simulink model "RT_01"  (R2018b)
settings: Solver=FixedStepAuto  StartTime=0.0  StopTime=40  FixedStep=0.01  RelTol=1e-3
undefined symbols (not defined in the file): circle, DiscIntNeverNeededParam, Measurement_Computing, National_Instruments, PCI, QUAD04
libraries: sldrtlib x25, simulink x8, simulink_extras x2
(part 1 of 2)
settings Model: ExtModeTrigDuration=120000  Creator=THIEN  LastModifiedBy=TMP
settings SolverCC: AutoInsertRateTranBlk=on  InsertRTBMode=Always
settings DataIOCC: LimitDataPoints=on  MaxDataPoints=25000  SaveFinalState=on  SaveFormat=StructureWithTime  DSMLogging=off  InspectSignalLogs=on  ReturnWorkspaceOutputs=on
settings HardwareCC: TargetLargestAtomicFloat=Float  TargetIntDivRoundTo=Zero  TargetEndianess=LittleEndian  TargetHWDeviceType=Intel->x86-32 (Windows32)
settings RTWCC: SystemTargetFile=sldrtert.tlc  TemplateMakefile=sldrtert.tmf  Description=Simulink Desktop Real-Time (ERT)  RTWCompilerOptimization=on
settings CodeAppCC: MaxIdLength=95
settings SimulinkDesktopRealTimeERTCC: TargetFcnLib=ansi_tfl_table_tmw.mat  TargetLibSuffix=_sldrt.lib  TargetPreCompLibLocation=C:\Program Files\MATLAB\R2018\toolbox\sldrt\lib\win64  GenFloatMathFcnCalls=NOT IN USE  TargetLangStandard=C99 (ISO)  CodeReplacementLibrary=None  UtilityFuncGeneration=Auto  MultiwordTypeDef=System defined  MultiwordLength=2048  DynamicStringBufferSize=256  GenerateFullHeader=on  InferredTypesCompatibility=off  GenerateSampleERTMain=off  GenerateTestInterfaces=off  ModelReferenceCompliant=on  ParMdlRefBuildCompliant=off  CompOptLevelCompliant=on  ConcurrentExecutionCompliant=off  IncludeMdlTerminateFcn=on  GeneratePreprocessorConditionals=Use local settings  CombineOutputUpdateFcns=off  CombineSignalStateStructs=off  GroupInternalDataByFunction=off  SuppressErrorStatus=off  IncludeFileDelimiter=Auto  ERTCustomFileBanners=off  SupportAbsoluteTime=on  LogVarNameModifier=rt_  MatFileLogging=off  MultiInstanceERTCode=off  CodeInterfacePackaging=Nonreusable function  PurelyIntegerCode=off  SupportNonFinite=on  SupportComplex=on  SupportContinuousTime=on  SupportNonInlinedSFcns=on  RemoveDisableFunc=off  RemoveResetFunc=off  SupportVariableSizeSignals=on  ParenthesesLevel=Nominal  CastingMode=Nominal  PreserveStateflowLocalDataDimensions=off  MATLABClassNameForMDSCustomization=Simulink.SoftwareTarget.TargetSpecificTriggerConfigurationBase  ModelStepFunctionPrototypeControlCompliant=off  CPPClassGenCompliant=off  AutosarCompliant=off  MDXCompliant=off  GRTInterface=off  GenerateAllocFcn=off  UseToolchainInfoCompliant=off  GenerateSharedConstants=on  CoderGroups=[]  AccessMethods=[]  LookupTableObjectStructAxisOrder=1,2,3,4,...  LUTObjectStructOrderExplicitValues=Size,Breakpoints,Table  LUTObjectStructOrderEvenSpacing=Size,Breakpoints,Table  ArrayLayout=Column-major  UnsupportedSFcnMsg=error  ERTHeaderFileRootName=$R$E  ERTSourceFileRootName=$R$E  ERTDataFileRootName=$R_data  GenerateASAP2=off  DSAsUniqueAccess=off  InlinedParameterPlacement=Hierarchical  TargetOS=BareBoardExample  MultiInstanceErrorCode=Error  RootIOFormat=Individual arguments  RTWCAPISignals=off  RTWCAPIParams=off  RTWCAPIStates=off  RTWCAPIRootIO=off  ERTSrcFileBannerTemplate=ert_code_template.cgt  ERTHdrFileBannerTemplate=ert_code_template.cgt  ERTDataSrcFileTemplate=ert_code_template.cgt  ERTDataHdrFileTemplate=ert_code_template.cgt  ERTCustomFileTemplate=example_file_process.tlc  EnableDataOwnership=off  SignalDisplayLevel=10  ParamTuneLevel=10  GlobalDataDefinition=Auto  DataDefinitionFile=global.c  GlobalDataReference=Auto  ERTFilePackagingFormat=Modular  RateTransitionBlockCode=Inline  DataReferenceFile=global.h  PreserveExpressionOrder=off  PreserveIfCondition=off  ConvertIfToSwitch=off  PreserveExternInFcnDecls=on  PreserveStaticInFcnDecls=on  SuppressUnreachableDefaultCases=off  EnableSignedLeftShifts=on  EnableSignedRightShifts=on  IndentStyle=K&R  IndentSize=2  NewlineStyle=Default  EnableUserReplacementTypes=off  MaxIdInt64=MAX_int64_T  MinIdInt64=MIN_int64_T  MaxIdUint64=MAX_uint64_T  MaxIdInt32=MAX_int32_T  MinIdInt32=MIN_int32_T  MaxIdUint32=MAX_uint32_T  MaxIdInt16=MAX_int16_T  MinIdInt16=MIN_int16_T  MaxIdUint16=MAX_uint16_T  MaxIdInt8=MAX_int8_T  MinIdInt8=MIN_int8_T  MaxIdUint8=MAX_uint8_T  BooleanTrueId=true  BooleanFalseId=false  MemSecPackage=--- None ---  MemSecDataConstants=Default  MemSecDataIO=Default  MemSecDataInternal=Default  MemSecDataParameters=Default  MemSecFuncInitTerm=Default  MemSecFuncExecute=Default  MemSecFuncSharedUtil=Default  GroupConstants=Default  GroupRootInputs=Default  GroupRootOutputs=Default  GroupInternal=Default  GroupParameters=Default  GroupDataTransfer=Default  GroupSharedLocalDataStores=Default  GroupInstanceSpecificParameters=Default  GroupModelData=Default  CCListing=off  RebuildAll=off  ExtMode=on  ExtModeTransport=0  ExtModeStaticAlloc=off  ExtModeStaticAllocSize=1000000  ExtModeTesting=off  ExtModeMexFile=sldrtext  ExtModeIntrfLevel=Level1

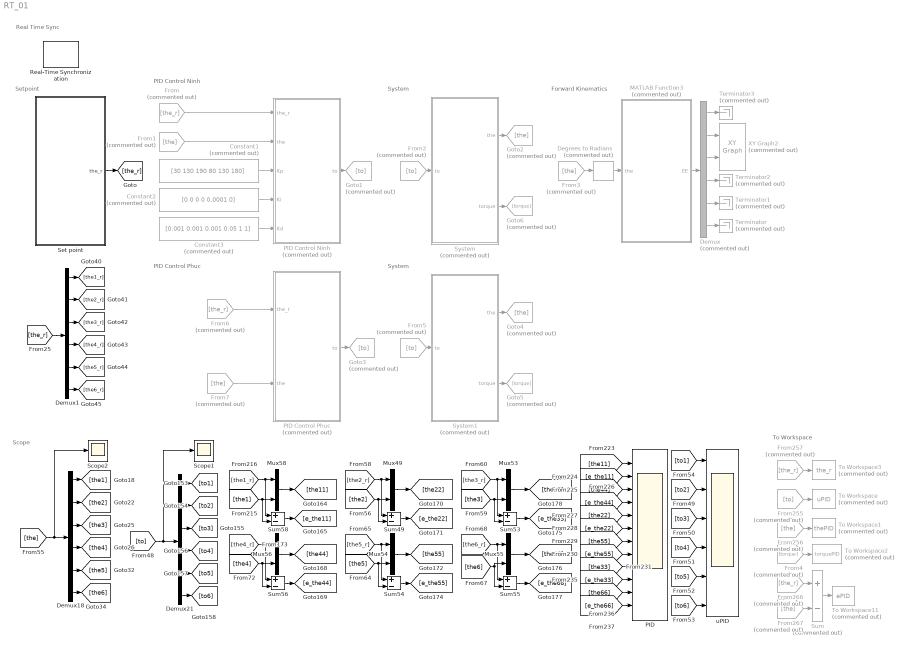
== system RT_01 ==
  note: Real Time Sync
  note: Forward Kinematics
  note: System
  note: PID Control Ninh
  note: Setpoint
  note: Scope
  note: System
  note: PID Control Phuc
  note: To Workspace
  Constant1 : Constant  Commented=on  Value=[30 130 190 80 130 180]
  Constant2 : Constant  Commented=on  Value=[0 0 0 0 0.0001 0]
  Constant3 : Constant  Commented=on  Value=[0.001 0.001 0.001 0.05 1 1]
  Degrees to Radians : simulink_extras/Transformations/Degrees to Radians  Commented=on
  Demux : Demux  Commented=on  Outputs=6
  Demux1 : Demux  Outputs=6
  Demux18 : Demux  Outputs=6
  Demux21 : Demux  Outputs=6
  From{,6,257,266} (4 alike) : From  Commented=on  GotoTag=the_r
  From{1,3,7,256,267} (5 alike) : From  Commented=on  GotoTag=the
  From2 : From  Commented=on  GotoTag=to
  From255 : From  Commented=on  GotoTag=to
  From4 : From  Commented=on  GotoTag=torque
  From5 : From  Commented=on  GotoTag=to
  Goto1 : Goto  Commented=on  GotoTag=to
  Goto2 : Goto  Commented=on  GotoTag=the
  Goto3 : Goto  Commented=on  GotoTag=to
  Goto4 : Goto  Commented=on  GotoTag=the
  Goto5 : Goto  Commented=on  GotoTag=torque
  Goto6 : Goto  Commented=on  GotoTag=torque
  MATLAB Function3 : MATLAB Function  Commented=on  TreatAsAtomicUnit=on
  Mux{49,53..56,58} (6 alike) : Mux  Inputs=2
  PID : Scope  NumInputPorts=12
  PID Control Ninh : Subsystem  Commented=on
  PID Control Phuc : Subsystem  Commented=on
  Real-Time Synchronization : sldrtlib/Real-Time Synchronization  SampleTime=0.01  MaxMissedTicks=10  ShowMissedTicks=off  YieldWhenWaiting=off
  Scope1 : Scope
  Scope2 : Scope
  Set point : Subsystem
  Sum : Sum  Commented=on  Inputs=+-
  Sum{49,53..56,58} (6 alike) : Sum  Inputs=+-
  System : Subsystem  Commented=on
  System1 : Subsystem  Commented=on
  Terminator{,1..3} (4 alike) : Terminator  Commented=on
  To Workspace : ToWorkspace  Commented=on  VariableName=uPID  SaveFormat=Structure With Time  SampleTime=-1
  To Workspace1 : ToWorkspace  Commented=on  VariableName=thePID  SaveFormat=Structure With Time  SampleTime=-1
  To Workspace11 : ToWorkspace  Commented=on  VariableName=ePID  SaveFormat=Structure With Time  SampleTime=-1
  To Workspace2 : ToWorkspace  Commented=on  VariableName=torquePID  SaveFormat=Structure With Time  SampleTime=-1
  To Workspace3 : ToWorkspace  Commented=on  VariableName=the_r  SaveFormat=Structure With Time  SampleTime=-1
  XY Graph2 : simulink/Sinks/XY Graph  Commented=on  xmin=-120  xmax=120  ymin=430  ymax=670  st=-1
  uPID : Scope  NumInputPorts=6
  wires:
  MATLAB Function3/1(EE) -> Demux/1
  Degrees to Radians/1 -> MATLAB Function3/1(the)
  Demux/2 -> XY Graph2/1
  Demux/3 -> XY Graph2/2
  Demux/6 -> Terminator/1
  Demux/5 -> Terminator1/1
  Demux/4 -> Terminator2/1
  Demux/1 -> Terminator3/1
  Constant1/1 -> PID Control Ninh/3(Kp)
  Constant3/1 -> PID Control Ninh/5(Kd)
  Constant2/1 -> PID Control Ninh/4(Ki)
  Set point/1(the_r) -> [the_r]
  From/1 -> PID Control Ninh/1(the_r)
  From1/1 -> PID Control Ninh/2(the)
  PID Control Ninh/1(to) -> Goto1/1
  From2/1 -> System/1(to)
  System/1(the) -> Goto2/1
  From3/1 -> Degrees to Radians/1
  [to2] -> uPID/2
  [to1] -> uPID/1
  [the22] -> PID/5
  [e_the55] -> PID/8
  [e_the66] -> PID/12
  Demux18/6 -> [the6]
  [to5] -> uPID/5
  [e_the22] -> PID/6
  [to3] -> uPID/3
  [the11] -> PID/1
  [the44] -> PID/3
  Mux53/1 -> [the33]
  Mux54/1 -> [the55]
  Sum53/1 -> [e_the33]
  [e_the44] -> PID/4
  [the66] -> PID/11
  Mux49/1 -> [the22]
  [the5] -> Mux54/2, Sum54/2
  Mux56/1 -> [the44]
  Sum58/1 -> [e_the11]
  Demux21/4 -> [to4]
  Sum55/1 -> [e_the66]
  [the1_r] -> Mux58/1, Sum58/1
  Demux18/5 -> [the5]
  [the3] -> Mux53/2, Sum53/2
  Sum49/1 -> [e_the22]
  [the1] -> Mux58/2, Sum58/2
  [the3_r] -> Mux53/1, Sum53/1
  Mux58/1 -> [the11]
  Sum54/1 -> [e_the55]
  [the5_r] -> Mux54/1, Sum54/1
  [the6] -> Mux55/2, Sum55/2
  Sum56/1 -> [e_the44]
  [to] -> Scope1/1, Demux21/1
  Demux21/3 -> [to3]
  [to4] -> uPID/4
  [the4] -> Sum56/2, Mux56/2
  Demux21/2 -> [to2]
  Demux21/6 -> [to6]
  Demux18/4 -> [the4]
  [the4_r] -> Sum56/1, Mux56/1
  Demux18/3 -> [the3]
  [e_the33] -> PID/10
  [e_the11] -> PID/2
  [the6_r] -> Sum55/1, Mux55/1
  [the2] -> Sum49/2, Mux49/2
  [to6] -> uPID/6
  Demux18/2 -> [the2]
  Demux21/5 -> [to5]
  [the33] -> PID/9
  Mux55/1 -> [the66]
  Demux18/1 -> [the1]
  [the55] -> PID/7
  Demux21/1 -> [to1]
  [the2_r] -> Sum49/1, Mux49/1
  Demux1/4 -> [the4_r]
  [the_r] -> Demux1/1
  Demux1/6 -> [the6_r]
  Demux1/3 -> [the3_r]
  Demux1/5 -> [the5_r]
  Demux1/1 -> [the1_r]
  Demux1/2 -> [the2_r]
  PID Control Phuc/1(to) -> Goto3/1
  From6/1 -> PID Control Phuc/1(the_r)
  From7/1 -> PID Control Phuc/2(the)
  System1/1(the) -> Goto4/1
  From5/1 -> System1/1(to)
  [the] -> Scope2/1, Demux18/1
  System1/2(torque) -> Goto5/1
  Sum/1 -> To Workspace11/1
  From266/1 -> Sum/1
  From257/1 -> To Workspace3/1
  From256/1 -> To Workspace1/1
  From267/1 -> Sum/2
  From255/1 -> To Workspace/1
  System/2(torque) -> Goto6/1
  From4/1 -> To Workspace2/1

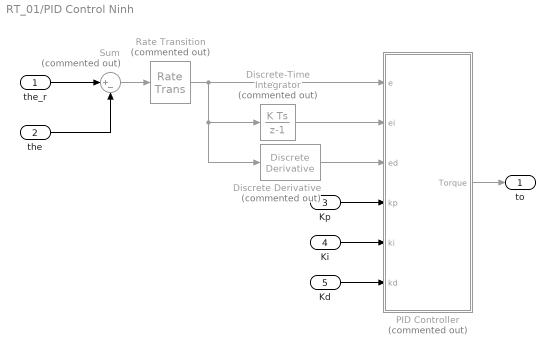
== system RT_01/PID Control Ninh ==
  the_r : Inport
  the : Inport  Port=2
  Kp : Inport  Port=3
  Ki : Inport  Port=4
  Kd : Inport  Port=5
  Discrete Derivative : simulink/Discrete/Discrete Derivative  Commented=on  gainval=1.0  ICPrevScaledInput=0.0  OutMin=[]  OutMax=[]  OutDataType=fixdt(1, 16)  OutScaling=2^-10  DoSatur=off
  Discrete-Time Integrator : DiscreteIntegrator  Commented=on  SampleTime=-1  ICPrevOutput=DiscIntNeverNeededParam  ICPrevScaledInput=DiscIntNeverNeededParam
  PID Controller : MATLAB Function  Commented=on  TreatAsAtomicUnit=on
  Rate Transition : RateTransition  Commented=on  OutPortSampleTime=0.01
  Sum : Sum  Commented=on  Inputs=|+-
  to : Outport
  wires:
  the/1 -> Sum/2
  Ki/1 -> PID Controller/5(ki)
  Discrete Derivative/1 -> PID Controller/3(ed)
  PID Controller/1(Torque) -> to/1
  Rate Transition/1 -> Discrete Derivative/1, Discrete-Time Integrator/1, PID Controller/1(e)
  Kp/1 -> PID Controller/4(kp)
  Kd/1 -> PID Controller/6(kd)
  Discrete-Time Integrator/1 -> PID Controller/2(ei)
  Sum/1 -> Rate Transition/1
  the_r/1 -> Sum/1

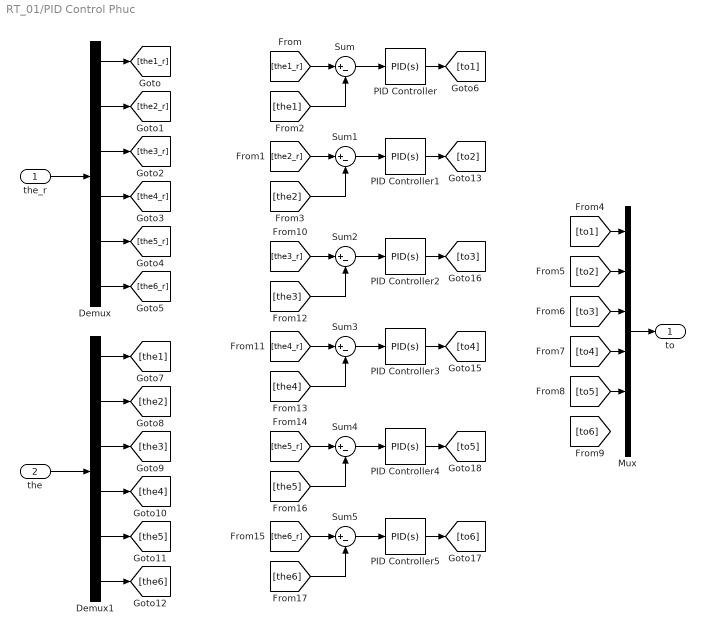
== system RT_01/PID Control Phuc ==
  the_r : Inport
  the : Inport  Port=2
  Demux : Demux  Outputs=6
  Demux1 : Demux  Outputs=6
  Mux : Mux  Inputs=6
  PID Controller : simulink/Continuous/PID Controller  Controller=PID  Form=Parallel  TimeDomain=Continuous-time  SampleTime=0.01  IntegratorMethod=Forward Euler  FilterMethod=Forward Euler  ControllerParametersSource=internal  P=90  I=0  D=4  UseFilter=on  N=100  TunerSelectOption=Transfer Function Based (PID Tuner App)  InitialConditionSource=internal  InitialConditionForIntegrator=0  InitialConditionForFilter=0  DifferentiatorICPrevScaledInput=0  ExternalReset=none  TrackingMode=off  Kt=1  LimitOutput=off  UpperSaturationLimit=inf  LowerSaturationLimit=-inf  LinearizeAsGain=on  AntiWindupMode=none  Kb=1  POutMin=[]  POutMax=[]  IOutMin=[]  IOutMax=[]  DOutMin=[]  DOutMax=[]  NOutMin=[]  NOutMax=[]  SumOutMin=[]  SumOutMax=[]  SaturationOutMin=[]  SaturationOutMax=[]  PParamMin=[]  PParamMax=[]  IParamMin=[]  IParamMax=[]  DParamMin=[]  DParamMax=[]  NParamMin=[]  NParamMax=[]  KbParamMin=[]  KbParamMax=[]  KtParamMin=[]  KtParamMax=[]  KbOutMin=[]  KbOutMax=[]  KtOutMin=[]  KtOutMax=[]  IntegratorOutMin=[]  IntegratorOutMax=[]  FilterOutMin=[]  FilterOutMax=[]  SumI1OutMin=[]  SumI1OutMax=[]  SumI2OutMin=[]  SumI2OutMax=[]  SumI3OutMin=[]  SumI3OutMax=[]  SumI4OutMin=[]  SumI4OutMax=[]  SumDOutMin=[]  SumDOutMax=[]  DifferentiatorOutMin=[]  DifferentiatorOutMax=[]  FilterDiffOutCoefMin=[]  FilterDiffOutCoefMax=[]  ReciprocalOutMin=[]  ReciprocalOutMax=[]  SumDenOutMin=[]  SumDenOutMax=[]  SumNumOutMin=[]  SumNumOutMax=[]  DivideOutMin=[]  DivideOutMax=[]  IntegratorContinuousStateAttributes=''  IntegratorStateMustResolveToSignalObject=off  IntegratorRTWStateStorageClass=Auto  FilterContinuousStateAttributes=''  FilterStateMustResolveToSignalObject=off  FilterRTWStateStorageClass=Auto  ParallelPVariant=InternalParameters  IdealPVariant=Disabled  IVariant=InternalParameters  DVariant=InternalParameters  IntegratorVariant=Continuous  SatVariant=Disabled  AWVariant=Passthrough  PCopyVariant=Disabled  TRVariant=Disabled  FdbkBlocksVariant=Forward  IdealPFdbkVariant=Disabled  SatFdbkVariant=Disabled  DerivativeFilterVariant=ContFilter  NVariant=InternalParameters  NCopyVariant=Disabled  FilterICVariant=InternalICsFilter  IntegratorICVariant=InternalICs  ExternalResetVariant=Disabled  TRSumVariant=Passthrough  SumFdbkVariant=Disabled  SumVariant=Sum_PID
  PID Controller1 : simulink/Continuous/PID Controller  Controller=PID  Form=Parallel  TimeDomain=Continuous-time  SampleTime=0.01  IntegratorMethod=Forward Euler  FilterMethod=Forward Euler  ControllerParametersSource=internal  P=220  I=0  D=12  UseFilter=on  N=100  TunerSelectOption=Transfer Function Based (PID Tuner App)  InitialConditionSource=internal  InitialConditionForIntegrator=0  InitialConditionForFilter=0  DifferentiatorICPrevScaledInput=0  ExternalReset=none  TrackingMode=off  Kt=1  LimitOutput=off  UpperSaturationLimit=inf  LowerSaturationLimit=-inf  LinearizeAsGain=on  AntiWindupMode=none  Kb=1  POutMin=[]  POutMax=[]  IOutMin=[]  IOutMax=[]  DOutMin=[]  DOutMax=[]  NOutMin=[]  NOutMax=[]  SumOutMin=[]  SumOutMax=[]  SaturationOutMin=[]  SaturationOutMax=[]  PParamMin=[]  PParamMax=[]  IParamMin=[]  IParamMax=[]  DParamMin=[]  DParamMax=[]  NParamMin=[]  NParamMax=[]  KbParamMin=[]  KbParamMax=[]  KtParamMin=[]  KtParamMax=[]  KbOutMin=[]  KbOutMax=[]  KtOutMin=[]  KtOutMax=[]  IntegratorOutMin=[]  IntegratorOutMax=[]  FilterOutMin=[]  FilterOutMax=[]  SumI1OutMin=[]  SumI1OutMax=[]  SumI2OutMin=[]  SumI2OutMax=[]  SumI3OutMin=[]  SumI3OutMax=[]  SumI4OutMin=[]  SumI4OutMax=[]  SumDOutMin=[]  SumDOutMax=[]  DifferentiatorOutMin=[]  DifferentiatorOutMax=[]  FilterDiffOutCoefMin=[]  FilterDiffOutCoefMax=[]  ReciprocalOutMin=[]  ReciprocalOutMax=[]  SumDenOutMin=[]  SumDenOutMax=[]  SumNumOutMin=[]  SumNumOutMax=[]  DivideOutMin=[]  DivideOutMax=[]  IntegratorContinuousStateAttributes=''  IntegratorStateMustResolveToSignalObject=off  IntegratorRTWStateStorageClass=Auto  FilterContinuousStateAttributes=''  FilterStateMustResolveToSignalObject=off  FilterRTWStateStorageClass=Auto  ParallelPVariant=InternalParameters  IdealPVariant=Disabled  IVariant=InternalParameters  DVariant=InternalParameters  IntegratorVariant=Continuous  SatVariant=Disabled  AWVariant=Passthrough  PCopyVariant=Disabled  TRVariant=Disabled  FdbkBlocksVariant=Forward  IdealPFdbkVariant=Disabled  SatFdbkVariant=Disabled  DerivativeFilterVariant=ContFilter  NVariant=InternalParameters  NCopyVariant=Disabled  FilterICVariant=InternalICsFilter  IntegratorICVariant=InternalICs  ExternalResetVariant=Disabled  TRSumVariant=Passthrough  SumFdbkVariant=Disabled  SumVariant=Sum_PID
  PID Controller2 : simulink/Continuous/PID Controller  Controller=PID  Form=Parallel  TimeDomain=Continuous-time  SampleTime=0.01  IntegratorMethod=Forward Euler  FilterMethod=Forward Euler  ControllerParametersSource=internal  P=270  I=0  D=12  UseFilter=on  N=100  TunerSelectOption=Transfer Function Based (PID Tuner App)  InitialConditionSource=internal  InitialConditionForIntegrator=0  InitialConditionForFilter=0  DifferentiatorICPrevScaledInput=0  ExternalReset=none  TrackingMode=off  Kt=1  LimitOutput=off  UpperSaturationLimit=inf  LowerSaturationLimit=-inf  LinearizeAsGain=on  AntiWindupMode=none  Kb=1  POutMin=[]  POutMax=[]  IOutMin=[]  IOutMax=[]  DOutMin=[]  DOutMax=[]  NOutMin=[]  NOutMax=[]  SumOutMin=[]  SumOutMax=[]  SaturationOutMin=[]  SaturationOutMax=[]  PParamMin=[]  PParamMax=[]  IParamMin=[]  IParamMax=[]  DParamMin=[]  DParamMax=[]  NParamMin=[]  NParamMax=[]  KbParamMin=[]  KbParamMax=[]  KtParamMin=[]  KtParamMax=[]  KbOutMin=[]  KbOutMax=[]  KtOutMin=[]  KtOutMax=[]  IntegratorOutMin=[]  IntegratorOutMax=[]  FilterOutMin=[]  FilterOutMax=[]  SumI1OutMin=[]  SumI1OutMax=[]  SumI2OutMin=[]  SumI2OutMax=[]  SumI3OutMin=[]  SumI3OutMax=[]  SumI4OutMin=[]  SumI4OutMax=[]  SumDOutMin=[]  SumDOutMax=[]  DifferentiatorOutMin=[]  DifferentiatorOutMax=[]  FilterDiffOutCoefMin=[]  FilterDiffOutCoefMax=[]  ReciprocalOutMin=[]  ReciprocalOutMax=[]  SumDenOutMin=[]  SumDenOutMax=[]  SumNumOutMin=[]  SumNumOutMax=[]  DivideOutMin=[]  DivideOutMax=[]  IntegratorContinuousStateAttributes=''  IntegratorStateMustResolveToSignalObject=off  IntegratorRTWStateStorageClass=Auto  FilterContinuousStateAttributes=''  FilterStateMustResolveToSignalObject=off  FilterRTWStateStorageClass=Auto  ParallelPVariant=InternalParameters  IdealPVariant=Disabled  IVariant=InternalParameters  DVariant=InternalParameters  IntegratorVariant=Continuous  SatVariant=Disabled  AWVariant=Passthrough  PCopyVariant=Disabled  TRVariant=Disabled  FdbkBlocksVariant=Forward  IdealPFdbkVariant=Disabled  SatFdbkVariant=Disabled  DerivativeFilterVariant=ContFilter  NVariant=InternalParameters  NCopyVariant=Disabled  FilterICVariant=InternalICsFilter  IntegratorICVariant=InternalICs  ExternalResetVariant=Disabled  TRSumVariant=Passthrough  SumFdbkVariant=Disabled  SumVariant=Sum_PID
  PID Controller3 : simulink/Continuous/PID Controller  Controller=PID  Form=Parallel  TimeDomain=Continuous-time  SampleTime=0.01  IntegratorMethod=Forward Euler  FilterMethod=Forward Euler  ControllerParametersSource=internal  P=110  I=0  D=6  UseFilter=on  N=100  TunerSelectOption=Transfer Function Based (PID Tuner App)  InitialConditionSource=internal  InitialConditionForIntegrator=0  InitialConditionForFilter=0  DifferentiatorICPrevScaledInput=0  ExternalReset=none  TrackingMode=off  Kt=1  LimitOutput=off  UpperSaturationLimit=inf  LowerSaturationLimit=-inf  LinearizeAsGain=on  AntiWindupMode=none  Kb=1  POutMin=[]  POutMax=[]  IOutMin=[]  IOutMax=[]  DOutMin=[]  DOutMax=[]  NOutMin=[]  NOutMax=[]  SumOutMin=[]  SumOutMax=[]  SaturationOutMin=[]  SaturationOutMax=[]  PParamMin=[]  PParamMax=[]  IParamMin=[]  IParamMax=[]  DParamMin=[]  DParamMax=[]  NParamMin=[]  NParamMax=[]  KbParamMin=[]  KbParamMax=[]  KtParamMin=[]  KtParamMax=[]  KbOutMin=[]  KbOutMax=[]  KtOutMin=[]  KtOutMax=[]  IntegratorOutMin=[]  IntegratorOutMax=[]  FilterOutMin=[]  FilterOutMax=[]  SumI1OutMin=[]  SumI1OutMax=[]  SumI2OutMin=[]  SumI2OutMax=[]  SumI3OutMin=[]  SumI3OutMax=[]  SumI4OutMin=[]  SumI4OutMax=[]  SumDOutMin=[]  SumDOutMax=[]  DifferentiatorOutMin=[]  DifferentiatorOutMax=[]  FilterDiffOutCoefMin=[]  FilterDiffOutCoefMax=[]  ReciprocalOutMin=[]  ReciprocalOutMax=[]  SumDenOutMin=[]  SumDenOutMax=[]  SumNumOutMin=[]  SumNumOutMax=[]  DivideOutMin=[]  DivideOutMax=[]  IntegratorContinuousStateAttributes=''  IntegratorStateMustResolveToSignalObject=off  IntegratorRTWStateStorageClass=Auto  FilterContinuousStateAttributes=''  FilterStateMustResolveToSignalObject=off  FilterRTWStateStorageClass=Auto  ParallelPVariant=InternalParameters  IdealPVariant=Disabled  IVariant=InternalParameters  DVariant=InternalParameters  IntegratorVariant=Continuous  SatVariant=Disabled  AWVariant=Passthrough  PCopyVariant=Disabled  TRVariant=Disabled  FdbkBlocksVariant=Forward  IdealPFdbkVariant=Disabled  SatFdbkVariant=Disabled  DerivativeFilterVariant=ContFilter  NVariant=InternalParameters  NCopyVariant=Disabled  FilterICVariant=InternalICsFilter  IntegratorICVariant=InternalICs  ExternalResetVariant=Disabled  TRSumVariant=Passthrough  SumFdbkVariant=Disabled  SumVariant=Sum_PID
  PID Controller4 : simulink/Continuous/PID Controller  Controller=PID  Form=Parallel  TimeDomain=Continuous-time  SampleTime=0.01  IntegratorMethod=Forward Euler  FilterMethod=Forward Euler  ControllerParametersSource=internal  P=150  I=0  D=4  UseFilter=on  N=100  TunerSelectOption=Transfer Function Based (PID Tuner App)  InitialConditionSource=internal  InitialConditionForIntegrator=0  InitialConditionForFilter=0  DifferentiatorICPrevScaledInput=0  ExternalReset=none  TrackingMode=off  Kt=1  LimitOutput=off  UpperSaturationLimit=inf  LowerSaturationLimit=-inf  LinearizeAsGain=on  AntiWindupMode=none  Kb=1  POutMin=[]  POutMax=[]  IOutMin=[]  IOutMax=[]  DOutMin=[]  DOutMax=[]  NOutMin=[]  NOutMax=[]  SumOutMin=[]  SumOutMax=[]  SaturationOutMin=[]  SaturationOutMax=[]  PParamMin=[]  PParamMax=[]  IParamMin=[]  IParamMax=[]  DParamMin=[]  DParamMax=[]  NParamMin=[]  NParamMax=[]  KbParamMin=[]  KbParamMax=[]  KtParamMin=[]  KtParamMax=[]  KbOutMin=[]  KbOutMax=[]  KtOutMin=[]  KtOutMax=[]  IntegratorOutMin=[]  IntegratorOutMax=[]  FilterOutMin=[]  FilterOutMax=[]  SumI1OutMin=[]  SumI1OutMax=[]  SumI2OutMin=[]  SumI2OutMax=[]  SumI3OutMin=[]  SumI3OutMax=[]  SumI4OutMin=[]  SumI4OutMax=[]  SumDOutMin=[]  SumDOutMax=[]  DifferentiatorOutMin=[]  DifferentiatorOutMax=[]  FilterDiffOutCoefMin=[]  FilterDiffOutCoefMax=[]  ReciprocalOutMin=[]  ReciprocalOutMax=[]  SumDenOutMin=[]  SumDenOutMax=[]  SumNumOutMin=[]  SumNumOutMax=[]  DivideOutMin=[]  DivideOutMax=[]  IntegratorContinuousStateAttributes=''  IntegratorStateMustResolveToSignalObject=off  IntegratorRTWStateStorageClass=Auto  FilterContinuousStateAttributes=''  FilterStateMustResolveToSignalObject=off  FilterRTWStateStorageClass=Auto  ParallelPVariant=InternalParameters  IdealPVariant=Disabled  IVariant=InternalParameters  DVariant=InternalParameters  IntegratorVariant=Continuous  SatVariant=Disabled  AWVariant=Passthrough  PCopyVariant=Disabled  TRVariant=Disabled  FdbkBlocksVariant=Forward  IdealPFdbkVariant=Disabled  SatFdbkVariant=Disabled  DerivativeFilterVariant=ContFilter  NVariant=InternalParameters  NCopyVariant=Disabled  FilterICVariant=InternalICsFilter  IntegratorICVariant=InternalICs  ExternalResetVariant=Disabled  TRSumVariant=Passthrough  SumFdbkVariant=Disabled  SumVariant=Sum_PID
  PID Controller5 : simulink/Continuous/PID Controller  Controller=PID  Form=Parallel  TimeDomain=Continuous-time  SampleTime=0.01  IntegratorMethod=Forward Euler  FilterMethod=Forward Euler  ControllerParametersSource=internal  P=200  I=0  D=6  UseFilter=on  N=100  TunerSelectOption=Transfer Function Based (PID Tuner App)  InitialConditionSource=internal  InitialConditionForIntegrator=0  InitialConditionForFilter=0  DifferentiatorICPrevScaledInput=0  ExternalReset=none  TrackingMode=off  Kt=1  LimitOutput=off  UpperSaturationLimit=inf  LowerSaturationLimit=-inf  LinearizeAsGain=on  AntiWindupMode=none  Kb=1  POutMin=[]  POutMax=[]  IOutMin=[]  IOutMax=[]  DOutMin=[]  DOutMax=[]  NOutMin=[]  NOutMax=[]  SumOutMin=[]  SumOutMax=[]  SaturationOutMin=[]  SaturationOutMax=[]  PParamMin=[]  PParamMax=[]  IParamMin=[]  IParamMax=[]  DParamMin=[]  DParamMax=[]  NParamMin=[]  NParamMax=[]  KbParamMin=[]  KbParamMax=[]  KtParamMin=[]  KtParamMax=[]  KbOutMin=[]  KbOutMax=[]  KtOutMin=[]  KtOutMax=[]  IntegratorOutMin=[]  IntegratorOutMax=[]  FilterOutMin=[]  FilterOutMax=[]  SumI1OutMin=[]  SumI1OutMax=[]  SumI2OutMin=[]  SumI2OutMax=[]  SumI3OutMin=[]  SumI3OutMax=[]  SumI4OutMin=[]  SumI4OutMax=[]  SumDOutMin=[]  SumDOutMax=[]  DifferentiatorOutMin=[]  DifferentiatorOutMax=[]  FilterDiffOutCoefMin=[]  FilterDiffOutCoefMax=[]  ReciprocalOutMin=[]  ReciprocalOutMax=[]  SumDenOutMin=[]  SumDenOutMax=[]  SumNumOutMin=[]  SumNumOutMax=[]  DivideOutMin=[]  DivideOutMax=[]  IntegratorContinuousStateAttributes=''  IntegratorStateMustResolveToSignalObject=off  IntegratorRTWStateStorageClass=Auto  FilterContinuousStateAttributes=''  FilterStateMustResolveToSignalObject=off  FilterRTWStateStorageClass=Auto  ParallelPVariant=InternalParameters  IdealPVariant=Disabled  IVariant=InternalParameters  DVariant=InternalParameters  IntegratorVariant=Continuous  SatVariant=Disabled  AWVariant=Passthrough  PCopyVariant=Disabled  TRVariant=Disabled  FdbkBlocksVariant=Forward  IdealPFdbkVariant=Disabled  SatFdbkVariant=Disabled  DerivativeFilterVariant=ContFilter  NVariant=InternalParameters  NCopyVariant=Disabled  FilterICVariant=InternalICsFilter  IntegratorICVariant=InternalICs  ExternalResetVariant=Disabled  TRSumVariant=Passthrough  SumFdbkVariant=Disabled  SumVariant=Sum_PID
  Sum{,1..5} (6 alike) : Sum  Inputs=|+-
  to : Outport
  wires:
  PID Controller/1 -> [to1]
  Sum/1 -> PID Controller/1
  PID Controller1/1 -> [to2]
  Demux/6 -> [the6_r]
  Demux/4 -> [the4_r]
  Demux/5 -> [the5_r]
  Demux/3 -> [the3_r]
  Demux/2 -> [the2_r]
  Demux/1 -> [the1_r]
  the_r/1 -> Demux/1
  [the1_r] -> Sum/1
  the/1 -> Demux1/1
  Demux1/1 -> [the1]
  Demux1/2 -> [the2]
  Demux1/3 -> [the3]
  Demux1/5 -> [the5]
  Demux1/4 -> [the4]
  Demux1/6 -> [the6]
  [the1] -> Sum/2
  Sum1/1 -> PID Controller1/1
  [the2_r] -> Sum1/1
  [the2] -> Sum1/2
  [to1] -> Mux/1
  [to2] -> Mux/2
  [to3] -> Mux/3
  [to4] -> Mux/4
  [to5] -> Mux/5
  [the4] -> Sum3/2
  [the4_r] -> Sum3/1
  Sum3/1 -> PID Controller3/1
  [the3] -> Sum2/2
  [the3_r] -> Sum2/1
  PID Controller3/1 -> [to4]
  Sum2/1 -> PID Controller2/1
  PID Controller2/1 -> [to3]
  PID Controller4/1 -> [to5]
  Sum4/1 -> PID Controller4/1
  PID Controller5/1 -> [to6]
  [the5_r] -> Sum4/1
  [the5] -> Sum4/2
  Sum5/1 -> PID Controller5/1
  [the6_r] -> Sum5/1
  [the6] -> Sum5/2
  Mux/1 -> to/1

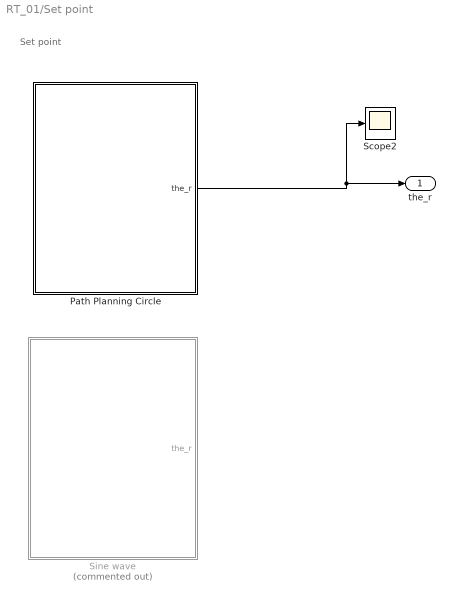
== system RT_01/Set point ==
  note: Set point
  Path Planning Circle : Subsystem
  Scope2 : Scope
  Sine wave : Subsystem  Commented=on
  the_r : Outport
  wires:
  Path Planning Circle/1(the_r) -> Scope2/1, the_r/1

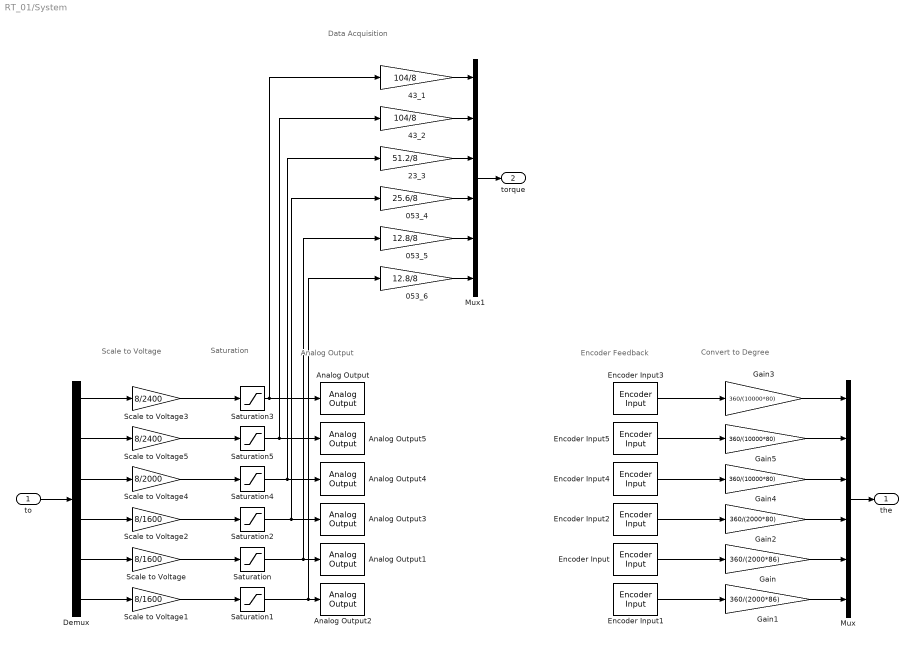
== system RT_01/System ==
  note: Data Acquisition
  note: Convert to Degree
  note: Encoder Feedback
  note: Analog Output
  note: Saturation
  note: Scale to Voltage
  to : Inport
  053_4 : Gain  Gain=25.6/8
  053_5 : Gain  Gain=12.8/8
  053_6 : Gain  Gain=12.8/8
  23_3 : Gain  Gain=51.2/8
  43_1 : Gain  Gain=104/8
  43_2 : Gain  Gain=104/8
  Analog Output : sldrtlib/Analog Output  SampleTime=0.01  MaxMissedTicks=10  ShowMissedTicks=off  YieldWhenWaiting=off  DrvName=National_Instruments/PCI-6713  DrvAddress=0  DrvOptions=[0 0]  Channels=7  RangeMode=1  VoltRange=1  InitialValue=0  FinalValue=0
      settings: AttributesFormatString=National Instruments\nPCI-6713 [0]  SourceProductName=Simulink Desktop Real-Time
  Analog Output1 : sldrtlib/Analog Output  SampleTime=0.01  MaxMissedTicks=10  ShowMissedTicks=off  YieldWhenWaiting=off  DrvName=National_Instruments/PCI-6713  DrvAddress=0  DrvOptions=[255 0]  Channels=5  RangeMode=1  VoltRange=1  InitialValue=0  FinalValue=0
      settings: AttributesFormatString=National Instruments\nPCI-6713 [0]  SourceProductName=Simulink Desktop Real-Time
  Analog Output2 : sldrtlib/Analog Output  SampleTime=0.01  MaxMissedTicks=10  ShowMissedTicks=off  YieldWhenWaiting=off  DrvName=National_Instruments/PCI-6713  DrvAddress=0  DrvOptions=[255 0]  Channels=6  RangeMode=1  VoltRange=1  InitialValue=0  FinalValue=0
      settings: AttributesFormatString=National Instruments\nPCI-6713 [0]  SourceProductName=Simulink Desktop Real-Time
  Analog Output3 : sldrtlib/Analog Output  SampleTime=0.01  MaxMissedTicks=10  ShowMissedTicks=off  YieldWhenWaiting=off  DrvName=National_Instruments/PCI-6713  DrvAddress=0  DrvOptions=[255 0]  Channels=4  RangeMode=1  VoltRange=1  InitialValue=0  FinalValue=0
      settings: AttributesFormatString=National Instruments\nPCI-6713 [0]  SourceProductName=Simulink Desktop Real-Time
  Analog Output4 : sldrtlib/Analog Output  SampleTime=0.01  MaxMissedTicks=10  ShowMissedTicks=off  YieldWhenWaiting=off  DrvName=National_Instruments/PCI-6713  DrvAddress=0  DrvOptions=[255 0]  Channels=3  RangeMode=1  VoltRange=1  InitialValue=0  FinalValue=0
      settings: AttributesFormatString=National Instruments\nPCI-6713 [0]  SourceProductName=Simulink Desktop Real-Time
  Analog Output5 : sldrtlib/Analog Output  SampleTime=0.01  MaxMissedTicks=10  ShowMissedTicks=off  YieldWhenWaiting=off  DrvName=National_Instruments/PCI-6713  DrvAddress=0  DrvOptions=[255 0]  Channels=2  RangeMode=1  VoltRange=1  InitialValue=0  FinalValue=0
      settings: AttributesFormatString=National Instruments\nPCI-6713 [0]  SourceProductName=Simulink Desktop Real-Time
  Demux : Demux  Outputs=6
  Encoder Input : sldrtlib/Encoder Input  SampleTime=0.01  MaxMissedTicks=10  ShowMissedTicks=off  YieldWhenWaiting=off  DrvName=Measurement_Computing/PCI-QUAD04  DrvAddress=1  DrvOptions=zeros(1,0)  Channels=3  QuadMode=3  IndexPulse=3  InputFilter=80000  DataType=1
      settings: AttributesFormatString=Measurement Computing\nPCI-QUAD04 [1]  SourceProductName=Simulink Desktop Real-Time
  Encoder Input1 : sldrtlib/Encoder Input  SampleTime=0.01  MaxMissedTicks=10  ShowMissedTicks=off  YieldWhenWaiting=off  DrvName=Measurement_Computing/PCI-QUAD04  DrvAddress=1  DrvOptions=zeros(1,0)  Channels=4  QuadMode=3  IndexPulse=3  InputFilter=80000  DataType=1
      settings: AttributesFormatString=Measurement Computing\nPCI-QUAD04 [1]  SourceProductName=Simulink Desktop Real-Time
  Encoder Input2 : sldrtlib/Encoder Input  SampleTime=0.01  MaxMissedTicks=10  ShowMissedTicks=off  YieldWhenWaiting=off  DrvName=Measurement_Computing/PCI-QUAD04  DrvAddress=2  DrvOptions=zeros(1,0)  Channels=4  QuadMode=3  IndexPulse=3  InputFilter=Inf  DataType=1
      settings: AttributesFormatString=Measurement Computing\nPCI-QUAD04 [2]  SourceProductName=Simulink Desktop Real-Time
  Encoder Input3 : sldrtlib/Encoder Input  SampleTime=0.01  MaxMissedTicks=10  ShowMissedTicks=off  YieldWhenWaiting=off  DrvName=Measurement_Computing/PCI-QUAD04  DrvAddress=2  DrvOptions=zeros(1,0)  Channels=1  QuadMode=3  IndexPulse=3  InputFilter=inf  DataType=1
      settings: AttributesFormatString=Measurement Computing\nPCI-QUAD04 [2]  SourceProductName=Simulink Desktop Real-Time
  Encoder Input4 : sldrtlib/Encoder Input  SampleTime=0.01  MaxMissedTicks=10  ShowMissedTicks=off  YieldWhenWaiting=off  DrvName=Measurement_Computing/PCI-QUAD04  DrvAddress=2  DrvOptions=zeros(1,0)  Channels=3  QuadMode=3  IndexPulse=3  InputFilter=inf  DataType=1
      settings: AttributesFormatString=Measurement Computing\nPCI-QUAD04 [2]  SourceProductName=Simulink Desktop Real-Time
  Encoder Input5 : sldrtlib/Encoder Input  SampleTime=0.01  MaxMissedTicks=10  ShowMissedTicks=off  YieldWhenWaiting=off  DrvName=Measurement_Computing/PCI-QUAD04  DrvAddress=2  DrvOptions=zeros(1,0)  Channels=2  QuadMode=3  IndexPulse=3  InputFilter=150000  DataType=1
      settings: AttributesFormatString=Measurement Computing\nPCI-QUAD04 [2]  SourceProductName=Simulink Desktop Real-Time
  Gain : Gain  Gain=360/(2000*86)
  Gain1 : Gain  Gain=360/(2000*86)
  Gain2 : Gain  Gain=360/(2000*80)
  Gain3 : Gain  Gain=360/(10000*80)
  Gain4 : Gain  Gain=360/(10000*80)
  Gain5 : Gain  Gain=360/(10000*80)
  Mux : Mux  Inputs=6
  Mux1 : Mux  Inputs=6
  Saturation{,1..5} (6 alike) : Saturate  UpperLimit=8  LowerLimit=-8
  Scale to Voltage : Gain  Gain=8/1600
  Scale to Voltage1 : Gain  Gain=8/1600
  Scale to Voltage2 : Gain  Gain=8/1600
  Scale to Voltage3 : Gain  Gain=8/2400
  Scale to Voltage4 : Gain  Gain=8/2000
  Scale to Voltage5 : Gain  Gain=8/2400
  the : Outport
  torque : Outport  Port=2
  wires:
  Saturation/1 -> 053_5/1, Analog Output1/1
  Encoder Input/1 -> Gain/1
  Scale to Voltage/1 -> Saturation/1
  Demux/5 -> Scale to Voltage/1
  Saturation1/1 -> 053_6/1, Analog Output2/1
  Encoder Input1/1 -> Gain1/1
  Scale to Voltage1/1 -> Saturation1/1
  Demux/6 -> Scale to Voltage1/1
  Demux/4 -> Scale to Voltage2/1
  Scale to Voltage2/1 -> Saturation2/1
  Encoder Input2/1 -> Gain2/1
  Saturation2/1 -> 053_4/1, Analog Output3/1
  Demux/1 -> Scale to Voltage3/1
  Saturation3/1 -> 43_1/1, Analog Output/1
  Encoder Input3/1 -> Gain3/1
  Scale to Voltage3/1 -> Saturation3/1
  Demux/3 -> Scale to Voltage4/1
  Saturation4/1 -> 23_3/1, Analog Output4/1
  Encoder Input4/1 -> Gain4/1
  Scale to Voltage4/1 -> Saturation4/1
  Saturation5/1 -> 43_2/1, Analog Output5/1
  Scale to Voltage5/1 -> Saturation5/1
  Encoder Input5/1 -> Gain5/1
  Demux/2 -> Scale to Voltage5/1
  to/1 -> Demux/1
  Gain/1 -> Mux/5
  Gain1/1 -> Mux/6
  Gain5/1 -> Mux/2
  Gain4/1 -> Mux/3
  Gain2/1 -> Mux/4
  Gain3/1 -> Mux/1
  Mux/1 -> the/1
  Mux1/1 -> torque/1
  053_5/1 -> Mux1/5
  053_6/1 -> Mux1/6
  053_4/1 -> Mux1/4
  23_3/1 -> Mux1/3
  43_2/1 -> Mux1/2
  43_1/1 -> Mux1/1

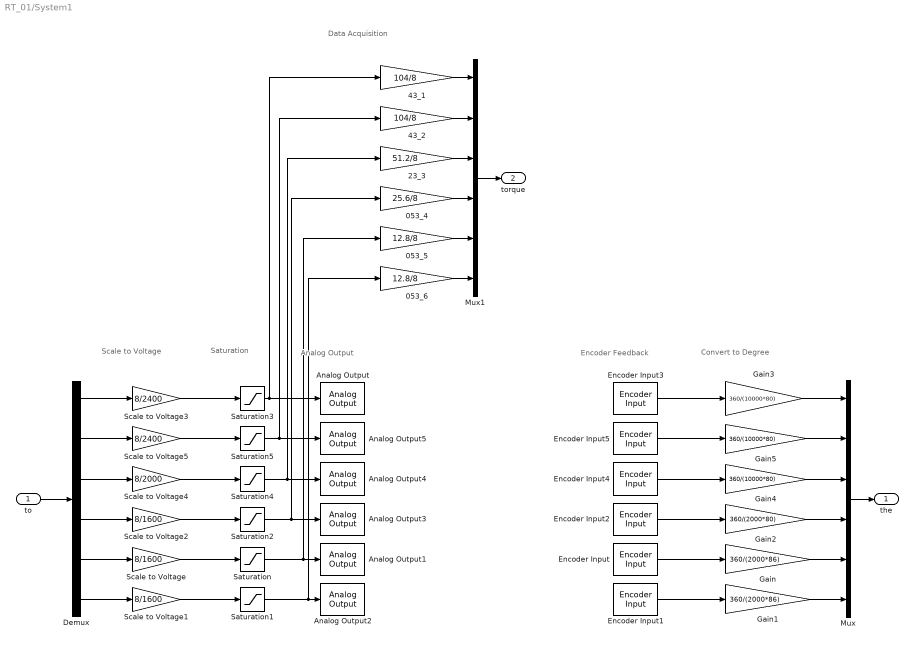
== system RT_01/System1 ==
  note: Scale to Voltage
  note: Saturation
  note: Analog Output
  note: Encoder Feedback
  note: Convert to Degree
  note: Data Acquisition
  to : Inport
  053_4 : Gain  Gain=25.6/8
  053_5 : Gain  Gain=12.8/8
  053_6 : Gain  Gain=12.8/8
  23_3 : Gain  Gain=51.2/8
  43_1 : Gain  Gain=104/8
  43_2 : Gain  Gain=104/8
  Analog Output : sldrtlib/Analog Output  SampleTime=0.01  MaxMissedTicks=10  ShowMissedTicks=off  YieldWhenWaiting=off  DrvName=National_Instruments/PCI-6713  DrvAddress=0  DrvOptions=[0 0]  Channels=7  RangeMode=1  VoltRange=1  InitialValue=0  FinalValue=0
      settings: AttributesFormatString=National Instruments\nPCI-6713 [0]  SourceProductName=Simulink Desktop Real-Time
  Analog Output1 : sldrtlib/Analog Output  SampleTime=0.01  MaxMissedTicks=10  ShowMissedTicks=off  YieldWhenWaiting=off  DrvName=National_Instruments/PCI-6713  DrvAddress=0  DrvOptions=[255 0]  Channels=5  RangeMode=1  VoltRange=1  InitialValue=0  FinalValue=0
      settings: AttributesFormatString=National Instruments\nPCI-6713 [0]  SourceProductName=Simulink Desktop Real-Time
  Analog Output2 : sldrtlib/Analog Output  SampleTime=0.01  MaxMissedTicks=10  ShowMissedTicks=off  YieldWhenWaiting=off  DrvName=National_Instruments/PCI-6713  DrvAddress=0  DrvOptions=[255 0]  Channels=6  RangeMode=1  VoltRange=1  InitialValue=0  FinalValue=0
      settings: AttributesFormatString=National Instruments\nPCI-6713 [0]  SourceProductName=Simulink Desktop Real-Time
  Analog Output3 : sldrtlib/Analog Output  SampleTime=0.01  MaxMissedTicks=10  ShowMissedTicks=off  YieldWhenWaiting=off  DrvName=National_Instruments/PCI-6713  DrvAddress=0  DrvOptions=[255 0]  Channels=4  RangeMode=1  VoltRange=1  InitialValue=0  FinalValue=0
      settings: AttributesFormatString=National Instruments\nPCI-6713 [0]  SourceProductName=Simulink Desktop Real-Time
  Analog Output4 : sldrtlib/Analog Output  SampleTime=0.01  MaxMissedTicks=10  ShowMissedTicks=off  YieldWhenWaiting=off  DrvName=National_Instruments/PCI-6713  DrvAddress=0  DrvOptions=[255 0]  Channels=3  RangeMode=1  VoltRange=1  InitialValue=0  FinalValue=0
      settings: AttributesFormatString=National Instruments\nPCI-6713 [0]  SourceProductName=Simulink Desktop Real-Time
  Analog Output5 : sldrtlib/Analog Output  SampleTime=0.01  MaxMissedTicks=10  ShowMissedTicks=off  YieldWhenWaiting=off  DrvName=National_Instruments/PCI-6713  DrvAddress=0  DrvOptions=[255 0]  Channels=2  RangeMode=1  VoltRange=1  InitialValue=0  FinalValue=0
      settings: AttributesFormatString=National Instruments\nPCI-6713 [0]  SourceProductName=Simulink Desktop Real-Time
  Demux : Demux  Outputs=6
  Encoder Input : sldrtlib/Encoder Input  SampleTime=0.01  MaxMissedTicks=10  ShowMissedTicks=off  YieldWhenWaiting=off  DrvName=Measurement_Computing/PCI-QUAD04  DrvAddress=1  DrvOptions=zeros(1,0)  Channels=3  QuadMode=3  IndexPulse=3  InputFilter=80000  DataType=1
      settings: AttributesFormatString=Measurement Computing\nPCI-QUAD04 [1]  SourceProductName=Simulink Desktop Real-Time
  Encoder Input1 : sldrtlib/Encoder Input  SampleTime=0.01  MaxMissedTicks=10  ShowMissedTicks=off  YieldWhenWaiting=off  DrvName=Measurement_Computing/PCI-QUAD04  DrvAddress=1  DrvOptions=zeros(1,0)  Channels=4  QuadMode=3  IndexPulse=3  InputFilter=100000  DataType=1
      settings: AttributesFormatString=Measurement Computing\nPCI-QUAD04 [1]  SourceProductName=Simulink Desktop Real-Time
  Encoder Input2 : sldrtlib/Encoder Input  SampleTime=0.01  MaxMissedTicks=10  ShowMissedTicks=off  YieldWhenWaiting=off  DrvName=Measurement_Computing/PCI-QUAD04  DrvAddress=2  DrvOptions=zeros(1,0)  Channels=4  QuadMode=3  IndexPulse=3  InputFilter=Inf  DataType=1
      settings: AttributesFormatString=Measurement Computing\nPCI-QUAD04 [2]  SourceProductName=Simulink Desktop Real-Time
  Encoder Input3 : sldrtlib/Encoder Input  SampleTime=0.01  MaxMissedTicks=10  ShowMissedTicks=off  YieldWhenWaiting=off  DrvName=Measurement_Computing/PCI-QUAD04  DrvAddress=2  DrvOptions=zeros(1,0)  Channels=1  QuadMode=3  IndexPulse=3  InputFilter=inf  DataType=1
      settings: AttributesFormatString=Measurement Computing\nPCI-QUAD04 [2]  SourceProductName=Simulink Desktop Real-Time
  Encoder Input4 : sldrtlib/Encoder Input  SampleTime=0.01  MaxMissedTicks=10  ShowMissedTicks=off  YieldWhenWaiting=off  DrvName=Measurement_Computing/PCI-QUAD04  DrvAddress=2  DrvOptions=zeros(1,0)  Channels=3  QuadMode=3  IndexPulse=3  InputFilter=inf  DataType=1
      settings: AttributesFormatString=Measurement Computing\nPCI-QUAD04 [2]  SourceProductName=Simulink Desktop Real-Time
  Encoder Input5 : sldrtlib/Encoder Input  SampleTime=0.01  MaxMissedTicks=10  ShowMissedTicks=off  YieldWhenWaiting=off  DrvName=Measurement_Computing/PCI-QUAD04  DrvAddress=2  DrvOptions=zeros(1,0)  Channels=2  QuadMode=3  IndexPulse=3  InputFilter=150000  DataType=1
      settings: AttributesFormatString=Measurement Computing\nPCI-QUAD04 [2]  SourceProductName=Simulink Desktop Real-Time
  Gain : Gain  Gain=360/(2000*86)
  Gain1 : Gain  Gain=360/(2000*86)
  Gain2 : Gain  Gain=360/(2000*80)
  Gain3 : Gain  Gain=360/(10000*80)
  Gain4 : Gain  Gain=360/(10000*80)
  Gain5 : Gain  Gain=360/(10000*80)
  Mux : Mux  Inputs=6
  Mux1 : Mux  Inputs=6
  Saturation{,1..5} (6 alike) : Saturate  UpperLimit=8  LowerLimit=-8
  Scale to Voltage : Gain  Gain=8/1600
  Scale to Voltage1 : Gain  Gain=8/1600
  Scale to Voltage2 : Gain  Gain=8/1600
  Scale to Voltage3 : Gain  Gain=8/2400
  Scale to Voltage4 : Gain  Gain=8/2000
  Scale to Voltage5 : Gain  Gain=8/2400
  the : Outport
  torque : Outport  Port=2
  wires:
  43_1/1 -> Mux1/1
  43_2/1 -> Mux1/2
  23_3/1 -> Mux1/3
  053_4/1 -> Mux1/4
  053_6/1 -> Mux1/6
  053_5/1 -> Mux1/5
  Mux1/1 -> torque/1
  Mux/1 -> the/1
  Gain3/1 -> Mux/1
  Gain2/1 -> Mux/4
  Gain4/1 -> Mux/3
  Gain5/1 -> Mux/2
  Gain1/1 -> Mux/6
  Gain/1 -> Mux/5
  to/1 -> Demux/1
  Demux/2 -> Scale to Voltage5/1
  Encoder Input5/1 -> Gain5/1
  Scale to Voltage5/1 -> Saturation5/1
  Saturation5/1 -> Analog Output5/1, 43_2/1
  Scale to Voltage4/1 -> Saturation4/1
  Encoder Input4/1 -> Gain4/1
  Saturation4/1 -> Analog Output4/1, 23_3/1
  Demux/3 -> Scale to Voltage4/1
  Scale to Voltage3/1 -> Saturation3/1
  Encoder Input3/1 -> Gain3/1
  Saturation3/1 -> Analog Output/1, 43_1/1
  Demux/1 -> Scale to Voltage3/1
  Saturation2/1 -> Analog Output3/1, 053_4/1
  Encoder Input2/1 -> Gain2/1
  Scale to Voltage2/1 -> Saturation2/1
  Demux/4 -> Scale to Voltage2/1
  Demux/6 -> Scale to Voltage1/1
  Scale to Voltage1/1 -> Saturation1/1
  Encoder Input1/1 -> Gain1/1
  Saturation1/1 -> Analog Output2/1, 053_6/1
  Demux/5 -> Scale to Voltage/1
  Scale to Voltage/1 -> Saturation/1
  Encoder Input/1 -> Gain/1
  Saturation/1 -> Analog Output1/1, 053_5/1

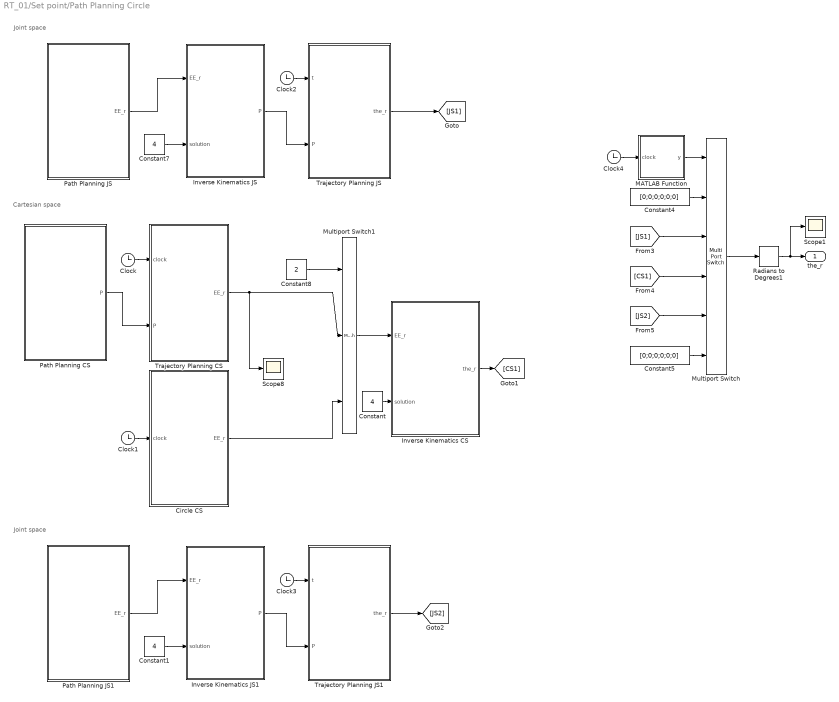
== system RT_01/Set point/Path Planning Circle ==
  note: Cartesian space
  note: Joint space
  note: Joint space
  Circle CS : MATLAB Function  TreatAsAtomicUnit=on
  Clock{,1..4} (5 alike) : Clock
  Constant : Constant  Value=4
  Constant1 : Constant  Value=4
  Constant4 : Constant  Value=[0;0;0;0;0;0]
  Constant5 : Constant  Value=[0;0;0;0;0;0]
  Constant7 : Constant  Value=4
  Constant8 : Constant  Value=2
  Inverse Kinematics CS : MATLAB Function  TreatAsAtomicUnit=on
  Inverse Kinematics JS : MATLAB Function  TreatAsAtomicUnit=on
  Inverse Kinematics JS1 : MATLAB Function  TreatAsAtomicUnit=on
  MATLAB Function : MATLAB Function  TreatAsAtomicUnit=on
  Multiport Switch : MultiPortSwitch  Inputs=5
  Multiport Switch1 : MultiPortSwitch  Inputs=2
  Path Planning CS : Subsystem
  Path Planning JS : Subsystem
  Path Planning JS1 : Subsystem
  Radians to Degrees1 : simulink_extras/Transformations/Radians to Degrees
  Scope1 : Scope
  Scope8 : Scope
  Trajectory Planning CS : MATLAB Function  TreatAsAtomicUnit=on
  Trajectory Planning JS : MATLAB Function  TreatAsAtomicUnit=on
  Trajectory Planning JS1 : MATLAB Function  TreatAsAtomicUnit=on
  the_r : Outport
  wires:
  Path Planning CS/1(P) -> Trajectory Planning CS/2(P)
  Constant7/1 -> Inverse Kinematics JS/2(solution)
  Clock1/1 -> Circle CS/1(clock)
  Clock2/1 -> Trajectory Planning JS/1(t)
  Constant8/1 -> Multiport Switch1/1
  Trajectory Planning JS/1(the_r) -> [JS1]
  Multiport Switch1/1 -> Inverse Kinematics CS/1(EE_r)
  Inverse Kinematics JS/1(P) -> Trajectory Planning JS/2(P)
  Constant/1 -> Inverse Kinematics CS/2(solution)
  Circle CS/1(EE_r) -> Multiport Switch1/3
  Path Planning JS/1(EE_r) -> Inverse Kinematics JS/1(EE_r)
  Trajectory Planning CS/1(EE_r) -> Scope8/1, Multiport Switch1/2
  Inverse Kinematics CS/1(the_r) -> [CS1]
  Clock/1 -> Trajectory Planning CS/1(clock)
  Path Planning JS1/1(EE_r) -> Inverse Kinematics JS1/1(EE_r)
  Inverse Kinematics JS1/1(P) -> Trajectory Planning JS1/2(P)
  Clock3/1 -> Trajectory Planning JS1/1(t)
  Constant1/1 -> Inverse Kinematics JS1/2(solution)
  Trajectory Planning JS1/1(the_r) -> [JS2]
  Clock4/1 -> MATLAB Function/1(clock)
  Constant4/1 -> Multiport Switch/2
  [JS1] -> Multiport Switch/3
  [CS1] -> Multiport Switch/4
  [JS2] -> Multiport Switch/5
  Constant5/1 -> Multiport Switch/6
  Radians to Degrees1/1 -> the_r/1, Scope1/1
  Multiport Switch/1 -> Radians to Degrees1/1
  MATLAB Function/1(y) -> Multiport Switch/1

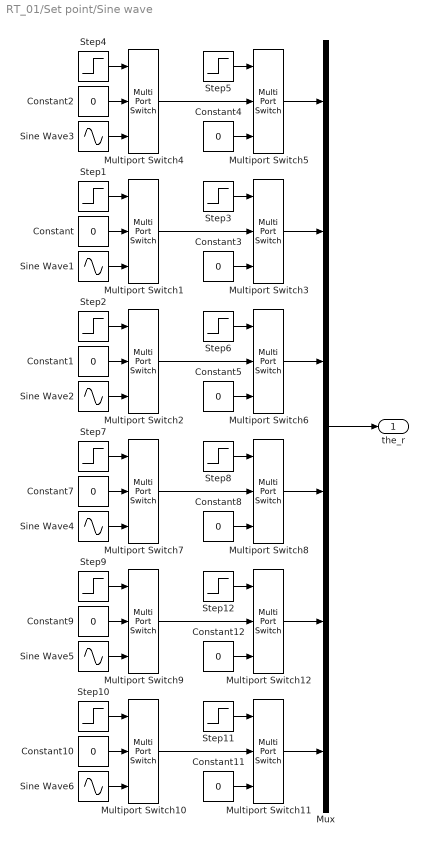
== system RT_01/Set point/Sine wave ==
  Constant{,1..5,7..12} (12 alike) : Constant  Value=0
  Multiport Switch{1..12} (12 alike) : MultiPortSwitch  Inputs=2
  Mux : Mux  Inputs=6
  Sine Wave{1..6} (6 alike) : Sin  Amplitude=30  Frequency=2*pi/10  SampleTime=0
  Step{1..2,4,7,9..10} (6 alike) : Step  Time=5  Before=1  After=2  SampleTime=0
  Step{3,5..6,8,11..12} (6 alike) : Step  Time=15  Before=1  After=2  SampleTime=0
  the_r : Outport
  wires:
  Constant1/1 -> Multiport Switch2/2
  Sine Wave2/1 -> Multiport Switch2/3
  Constant11/1 -> Multiport Switch11/3
  Multiport Switch3/1 -> Mux/2
  Constant5/1 -> Multiport Switch6/3
  Multiport Switch2/1 -> Multiport Switch6/2
  Step7/1 -> Multiport Switch7/1
  Constant/1 -> Multiport Switch1/2
  Multiport Switch7/1 -> Multiport Switch8/2
  Step9/1 -> Multiport Switch9/1
  Multiport Switch8/1 -> Mux/4
  Sine Wave6/1 -> Multiport Switch10/3
  Sine Wave5/1 -> Multiport Switch9/3
  Constant3/1 -> Multiport Switch3/3
  Multiport Switch10/1 -> Multiport Switch11/2
  Constant10/1 -> Multiport Switch10/2
  Step10/1 -> Multiport Switch10/1
  Multiport Switch9/1 -> Multiport Switch12/2
  Multiport Switch1/1 -> Multiport Switch3/2
  Multiport Switch11/1 -> Mux/6
  Multiport Switch4/1 -> Multiport Switch5/2
  Step2/1 -> Multiport Switch2/1
  Constant4/1 -> Multiport Switch5/3
  Step4/1 -> Multiport Switch4/1
  Constant8/1 -> Multiport Switch8/3
  Multiport Switch12/1 -> Mux/5
  Constant2/1 -> Multiport Switch4/2
  Step5/1 -> Multiport Switch5/1
  Step11/1 -> Multiport Switch11/1
  Sine Wave3/1 -> Multiport Switch4/3
  Constant7/1 -> Multiport Switch7/2
  Step8/1 -> Multiport Switch8/1
  Sine Wave4/1 -> Multiport Switch7/3
  Step3/1 -> Multiport Switch3/1
  Step12/1 -> Multiport Switch12/1
  Constant9/1 -> Multiport Switch9/2
  Step1/1 -> Multiport Switch1/1
  Step6/1 -> Multiport Switch6/1
  Constant12/1 -> Multiport Switch12/3
  Sine Wave1/1 -> Multiport Switch1/3
  Multiport Switch5/1 -> Mux/1
  Multiport Switch6/1 -> Mux/3
  Mux/1 -> the_r/1

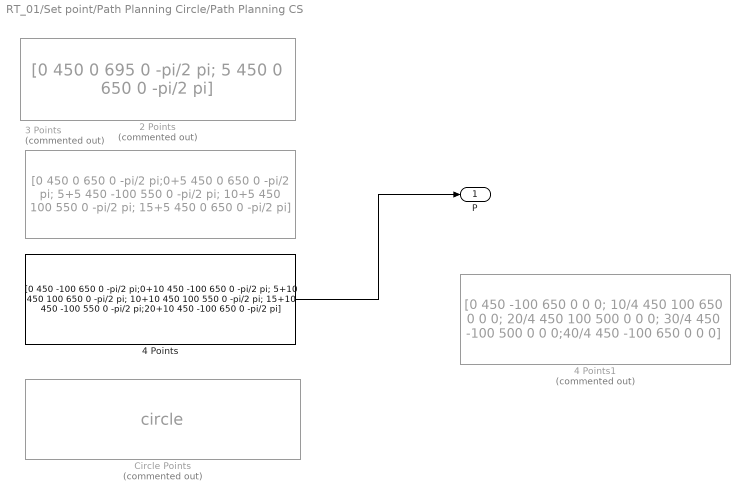
== system RT_01/Set point/Path Planning Circle/Path Planning CS ==
  2 Points : Constant  Commented=on  Value=[0 450 0 695 0 -pi/2 pi; 5 450 0 650 0 -pi/2 pi]
  3 Points : Constant  Commented=on  Value=[0 450 0 650 0 -pi/2 pi;0+5 450 0 650 0 -pi/2 pi; 5+5 450 -100 550 0 -pi/2 pi; 10+5 450 100 550 0 -pi/2 pi; 15+5 450 0 650 0 -pi/2 pi]
  4 Points : Constant  Value=[0 450 -100 650 0 -pi/2 pi;0+10 450 -100 650 0 -pi/2 pi; 5+10 450 100 650 0 -pi/2 pi; 10+10 450 100 550 0 -pi/2 pi; 15+10 450 -100 550 0 -pi/2 pi;20+10 450 -100 650 0 -pi/2 pi]
  4 Points1 : Constant  Commented=on  Value=[0 450 -100 650 0 0 0; 10/4 450 100 650 0 0 0; 20/4 450 100 500 0 0 0; 30/4 450 -100 500 0 0 0;40/4 450 -100 650 0 0 0]
  Circle Points : Constant  Commented=on  Value=circle
  P : Outport
  wires:
  4 Points/1 -> P/1

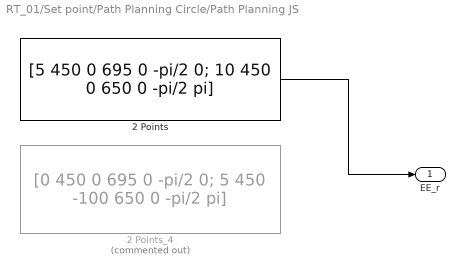
== system RT_01/Set point/Path Planning Circle/Path Planning JS ==
  2 Points : Constant  Value=[5 450 0 695 0 -pi/2 0; 10 450 0 650 0 -pi/2 pi]
  2 Points_4 : Constant  Commented=on  Value=[0 450 0 695 0 -pi/2 0; 5 450 -100 650 0 -pi/2 pi]
  EE_r : Outport
  wires:
  2 Points/1 -> EE_r/1

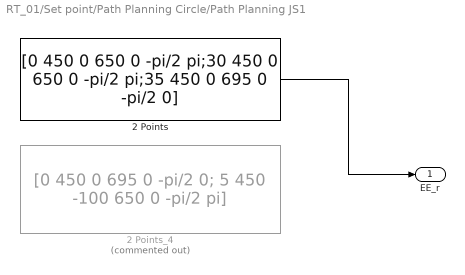
== system RT_01/Set point/Path Planning Circle/Path Planning JS1 ==
  2 Points : Constant  Value=[0 450 0 650 0 -pi/2 pi;30 450 0 650 0 -pi/2 pi;35 450 0 695 0 -pi/2 0]
  2 Points_4 : Constant  Commented=on  Value=[0 450 0 695 0 -pi/2 0; 5 450 -100 650 0 -pi/2 pi]
  EE_r : Outport
  wires:
  2 Points/1 -> EE_r/1

== matlab function RT_01/Set point/Path Planning Circle/Inverse Kinematics CS ==
  data: EE_r input; the_r output; solution input
function the_r  = IK_6DOF(EE_r,solution)
a1=75; a2=270; a3=90; d1=335; d4=295; d7=80;
emt = zeros(8,6);
m = 0;
px = EE_r(1);
py = EE_r(2);
pz = EE_r(3);
roll = EE_r(4);
pitch = EE_r(5);
yaw =  EE_r(6);
r11 = cos(yaw)*cos(pitch);
r21 = sin(yaw)*cos(pitch);
r31 = -sin(pitch);
r12 = cos(yaw)*sin(pitch)*sin(roll) - sin(yaw)*cos(roll);
r22 = sin(yaw)*sin(pitch)*sin(roll) + cos(yaw)*cos(roll);
r32 = cos(pitch)*sin(roll);
r13 = cos(yaw)*sin(pitch)*cos(roll) + sin(yaw)*sin(roll);
r23 = sin(yaw)*sin(pitch)*cos(roll) - cos(yaw)*sin(roll);
r33 = cos(pitch)*cos(roll);
% r11 = 1;
% r22 = 0;
% r33 = 0;
% r12 = 0;
% r21 = 0;
% r13 = 0;
% r31 = 0;
% r23 = -1;
% r32 = 1;
%% Inverse Kinematics
% Find the1
a_1 = py - r23*d7;
b_1 = - px + r13*d7;
d_1 = 0;
the11 = basic_01(a_1,b_1,d_1);
for i = 1:2
    % Find the2
    u = cos(the11(i))*(px-d7*r13) + sin(the11(i))*(py-r23*d7) - a1;
    v = pz - d1 - r33*d7;
    a_2 = v;
    b_2 = u;
    d_2 = (a3^2+d4^2-u^2-v^2-a2^2)/(-2*a2);
    if a_2*a_2 + b_2*b_2 - d_2*d_2 >=0
        the22 = basic_01(a_2,b_2,d_2);
    else
        continue;
    end
    for j = 1:2
        % Find the3
        a_3 = a3;
        b_3 = d4;
        c_3 = u*sin(the22(j)) + v*cos(the22(j)) - a2;
        d_3 = u*cos(the22(j)) - v*sin(the22(j));
        the33 = basic_02(a_3,b_3,c_3,d_3);
        
        % Find the5
        c5 = (r13*cos(the11(i))*cos(the22(j)) - r33*sin(the22(j)) + r23*cos(the22(j))*sin(the11(i)))*cos(the33) - (r33*cos(the22(j)) + r13*cos(the11(i))*sin(the22(j)) + r23*sin(the11(i))*sin(the22(j)))*sin(the33);
        if 1*1 + 0*0 - c5*c5 >=0
            the55 = basic_01(1,0,c5);
        else
            continue;
        end
        for k = 1:2
            % Find the4
            m = m+1;
            s4 = (r23*cos(the11(i)) - r13*sin(the11(i)))/(sin(the55(k)));
            c4 = (r33*cos(the22(j)) + r13*cos(the11(i))*sin(the22(j)) + r23*sin(the11(i))*sin(the22(j)) + sin(the33)*cos(the55(k))) / (-cos(the33)*sin(the55(k)));
            the44 = atan2(s4,c4);
            
            % Find the6
            a_6 = r21*cos(the11(i)) - r11*sin(the11(i));
            b_6 = r22*cos(the11(i)) - r12*sin(the11(i));
            c_6 = -sin(the44)*cos(the55(k));
            d_6 = cos(the44);
            the66 = basic_02(a_6,b_6,c_6,-d_6);
            emt(m,:)=[the11(i),the22(j),the33,the44,the55(k),the66];
        end
    end
end
% the = emt(solution,:);
the1 = emt(solution,1);
the2 = emt(solution,2);
the3 = emt(solution,3);
the4 = emt(solution,4);
the5 = emt(solution,5);
the6 = emt(solution,6);
the_r = [the1;the2;the3;the4;the5;the6];
end

function x = basic_01(a, b, d) % a*cos(x) + b*sin(x) = d
    anp = atan2(b, a);
    
    x1 = anp + atan2(sqrt(a*a + b*b - d*d), d);
    x2 = anp + atan2(-sqrt(a*a + b*b - d*d), d);
    x = [x1; x2];
end   

function x = basic_02(a, b, c, d) 
    % a*cos(x) - b*sin(x) = c
    % b*cos(x) + a*sin(x) = d
    sin = (d - b*c/a) / (b^2/a + a);
    cos = (c + b*d/a) / (b^2/a + a);
    x = atan2(sin,cos);
end

== matlab function RT_01/PID Control Ninh/PID Controller ==
  data: e input; ei input; Torque output; ed input; kp input; ki input; kd input
function Torque = PID(e,ei,ed,kp,ki,kd)
kp_ = diag(kp);
ki_ = diag(ki);
kd_ = diag(kd);
Torque = kp_*e + ki_*ei + kd_*ed;
